simulink model "darko_control_lineaire_lqi_vol"  (R2020b)
settings: Solver=VariableStepAuto  StartTime=0.0  StopTime=1  RelTol=1e-3
values from neighbouring files (symbols this model uses):
  initial_state = [p_; v_; q_; omega_]    [main_linearisation_vol.m]
  u_eq = [trim(1);trim(1);trim(2);trim(2)]    [main_linearisation_vol.m]
  v_initial = [v_trim; 0; 0]    [main_linearisation_vol.m]
  x_eq = [p_initial; v_initial; q_initial; omega_initial]    [main_linearisation_vol.m]
undefined symbols (not defined in the file or in its folder): K_complet_i
libraries: simulink_extras x3, sharedtransform x1
settings Model: Creator=florian  LastModifiedBy=florian

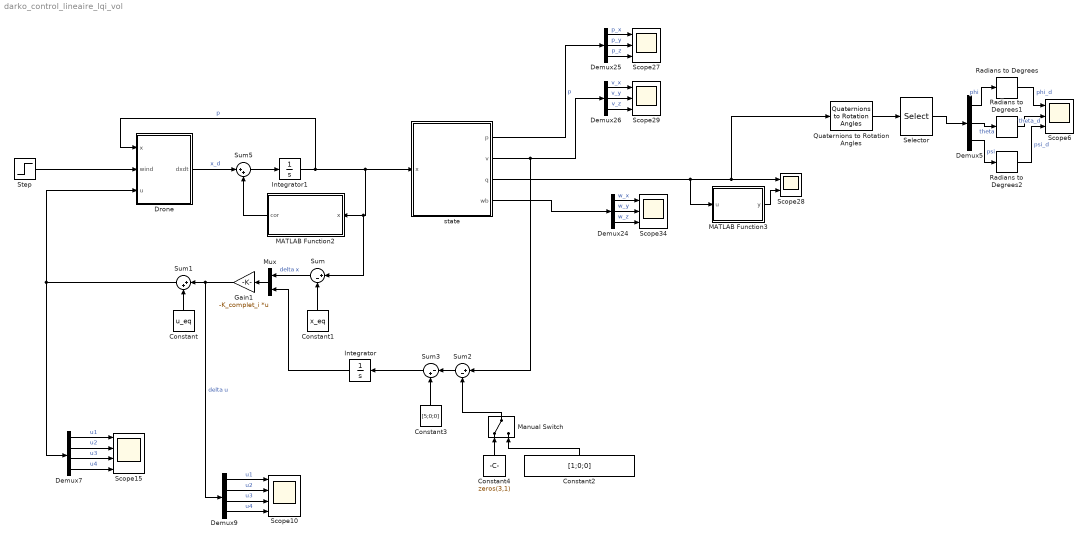
== system darko_control_lineaire_lqi_vol ==
  Constant : Constant  Value=u_eq
  Constant1 : Constant  Value=x_eq
  Constant2 : Constant  Value=[1;0;0]
  Constant3 : Constant  Value=[5;0;0]
  Constant4 : Constant  Value=zeros(3,1)
  Demux{5,24..26} (4 alike) : Demux  Outputs=3
  Demux7 : Demux
  Demux9 : Demux
  Drone : MATLAB Function  TreatAsAtomicUnit=on
  Gain1 : Gain  Gain=-K_complet_i  Multiplication=Matrix(K*u) (u vector)
  Integrator : Integrator  InitialCondition=v_initial
  Integrator1 : Integrator  InitialCondition=initial_state
  MATLAB Function2 : MATLAB Function  TreatAsAtomicUnit=on
  MATLAB Function3 : MATLAB Function  TreatAsAtomicUnit=on
  Manual Switch : ManualSwitch
  Mux : Mux  Inputs=2
  Quaternions to Rotation Angles : sharedtransform/Quaternions to Rotation Angles  rotationOrder=ZXY  aMode=aMode
      settings: SourceProductBaseCode=AE,PW,MT,UV,VE,VP
  Radians to Degrees : simulink_extras/Transformations/Radians to Degrees
  Radians to Degrees1 : simulink_extras/Transformations/Radians to Degrees
  Radians to Degrees2 : simulink_extras/Transformations/Radians to Degrees
  Scope10 : Scope  NumInputPorts=4
  Scope15 : Scope  NumInputPorts=4
  Scope{6,27,29,34} (4 alike) : Scope  NumInputPorts=3
  Scope28 : Scope  NumInputPorts=2
  Selector : Selector  InputPortWidth=3  IndexOptions=Index vector (dialog)  Indices=[2 3 1]  OutputSizes=1
  Step : Step  Time=10  Before=[0;0;0]  After=[0;0;0]  SampleTime=0
  Sum : Sum  Inputs=|+-
  Sum1 : Sum  Inputs=|++
  Sum2 : Sum  Inputs=|+-
  Sum3 : Sum  Inputs=|-+
  Sum5 : Sum  Inputs=|++
  state : MATLAB Function  TreatAsAtomicUnit=on
  wires:
  Sum5/1 -> Integrator1/1
  MATLAB Function2/1(cor) -> Sum5/2
  Drone/1(dxdt) -> Sum5/1  "x_d"
  Integrator1/1 -> Drone/1(x), state/1(x), Sum/1, MATLAB Function2/1(x)  "p"
  Demux25/3 -> Scope27/3  "p_z"
  Demux26/2 -> Scope29/2  "v_y"
  Demux24/1 -> Scope34/1  "w_x"
  MATLAB Function3/1(y) -> Scope28/2
  Demux25/1 -> Scope27/1  "p_x"
  state/4(wb) -> Demux24/1
  Demux24/2 -> Scope34/2  "w_y"
  Demux24/3 -> Scope34/3  "w_z"
  state/2(v) -> Sum2/1, Demux26/1
  Demux25/2 -> Scope27/2  "p_y"
  Demux26/3 -> Scope29/3  "v_z"
  Demux26/1 -> Scope29/1  "v_x"
  Gain1/1 -> Demux9/1, Sum1/1  "delta u"
  Sum1/1 -> Demux7/1, Drone/3(u)
  Constant/1 -> Sum1/2
  Constant1/1 -> Sum/2
  Demux7/3 -> Scope15/3  "u3"
  Demux7/4 -> Scope15/4  "u4"
  Demux7/1 -> Scope15/1  "u1"
  Demux7/2 -> Scope15/2  "u2"
  Demux9/3 -> Scope10/3  "u3"
  Demux9/4 -> Scope10/4  "u4"
  Demux9/1 -> Scope10/1  "u1"
  Demux9/2 -> Scope10/2  "u2"
  Step/1 -> Drone/2(wind)
  Sum3/1 -> Integrator/1
  Constant3/1 -> Sum3/2
  Mux/1 -> Gain1/1
  Integrator/1 -> Mux/2
  Sum/1 -> Mux/1  "delta x"
  Selector/1 -> Demux5/1
  Demux5/2 -> Radians to Degrees1/1  "theta"
  Quaternions to Rotation Angles/1 -> Selector/1
  state/3(q) -> MATLAB Function3/1(u), Quaternions to Rotation Angles/1, Scope28/1
  Demux5/1 -> Radians to Degrees/1  "phi"
  Radians to Degrees/1 -> Scope6/1  "phi_d"
  Radians to Degrees1/1 -> Scope6/2  "theta_d"
  Demux5/3 -> Radians to Degrees2/1  "psi"
  Radians to Degrees2/1 -> Scope6/3  "psi_d"
  state/1(p) -> Demux25/1  "p"
  Constant2/1 -> Manual Switch/2
  Constant4/1 -> Manual Switch/1
  Manual Switch/1 -> Sum2/2
  Sum2/1 -> Sum3/1

== matlab function darko_control_lineaire_lqi_vol/Drone ==
  data: x input; wind input; u input; dxdt output; drone parameter
function dxdt  = drone(x,wind, u, drone)

%% physical constants
% gravity
g = drone.G;
% vehicle mass
m = drone.MASS;
% vehicle inertia matrix
J = drone.INERTIA; % [3x3 real symmetric] in body axis

%% state demultiplexing
% p = x(1:3);
v = x(4:6);
q  = x(7:10);
wb = x(11:13);

Rq = q2dcm(q);

[Fp, Mp] = external_force_moment(x, u, wind, drone);

% position
dpdt = v;

% kinematics
dvdt =  -[0;0;g] + (1/m)*Rq*drone.Fb*u + (1/m)*Rq*Fp; 

%% quaternion derivative
eta = q(1);
eps = q(2:4);

dqdt = (1/2)*[-eps'; eta*eye(3) + skew_sym(eps)]*wb;

%% angular velocity derivative
% kinematics
dwdt = -J\cross(wb, J*wb) + J\(drone.Mb*u) + J\Mp;


%% derivative multiplexing
dxdt = [dpdt; dvdt; dqdt; dwdt] ;

== matlab function darko_control_lineaire_lqi_vol/MATLAB Function2 ==
  data: x input; cor output
function cor  = fcn(x)
%#codegen
q  = x(7:10);
n = norm(q);
mismatch = 1-n;
cor = [0;0;0; 0;0;0; mismatch*q; 0;0;0];

== matlab function darko_control_lineaire_lqi_vol/MATLAB Function3 ==
  data: u input; y output
function y = fcn(u)
%#codegen

y = norm(u);

== matlab function darko_control_lineaire_lqi_vol/state ==
  data: x input; p output; v output; q output; wb output
function [p, v, q, wb] = demux(x)
%#codegen

p = x(1:3);
v = x(4:6);
q  = x(7:10);
wb = x(11:13);
